simulink model "untitled"  (R2015a)
settings: Solver=ode3  StartTime=0.0  StopTime=40  FixedStep=0.2  RelTol=1e-3
settings Model: Creator=Caroline  LastModifiedBy=Caroline

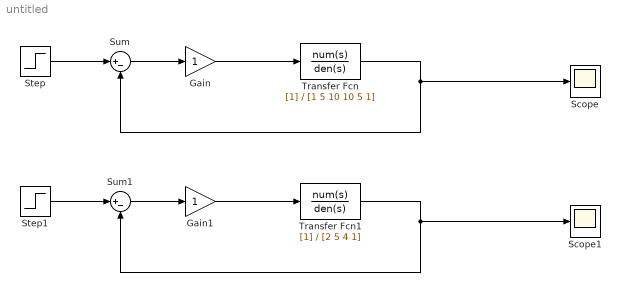
== system untitled ==
  Gain : Gain
  Gain1 : Gain
  Scope : Scope
      settings: TimeRange=20  MaxDataPoints=10000
  Scope1 : Scope
      settings: TimeRange=20  MaxDataPoints=10000
  Step : Step  SampleTime=0.2
  Step1 : Step  SampleTime=0.2
  Sum : Sum  Inputs=|+-
  Sum1 : Sum  Inputs=|+-
  Transfer Fcn : TransferFcn  Denominator=[1 5 10 10 5 1]
  Transfer Fcn1 : TransferFcn  Denominator=[2 5 4 1]
  wires:
  Step/1 -> Sum/1
  Sum/1 -> Gain/1
  Gain/1 -> Transfer Fcn/1
  Transfer Fcn/1 -> Sum/2, Scope/1
  Step1/1 -> Sum1/1
  Sum1/1 -> Gain1/1
  Gain1/1 -> Transfer Fcn1/1
  Transfer Fcn1/1 -> Sum1/2, Scope1/1
